simulink model "tank2"  (Simulink 7.3)
settings: Solver=ode45  StartTime=0.0  StopTime=20.0  RelTol=1e-3
undefined symbols (not defined in the file or in its folder): DiscIntNeverNeededParam
libraries: simulink x1
settings Model: Creator=nmd01  LastModifiedBy=nmd01

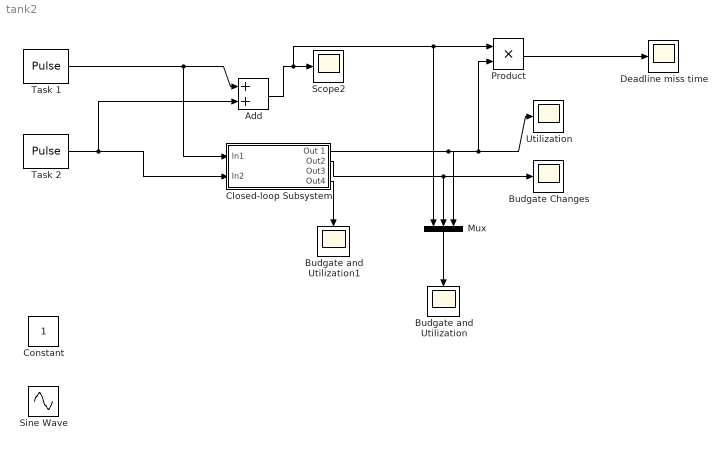
== system tank2 ==
  Add : Sum  OutDataType=fixdt(1, 16)  OutScaling=2^-10
  Budgate Changes : Scope
  Budgate and Utilization : Scope
      settings: TimeRange=200  YMin=0  YMax=30  SaveName=ScopeData3
  Budgate and Utilization1 : Scope
      settings: TimeRange=200  YMin=0  YMax=30
  Closed-loop Subsystem : Subsystem
  Constant : Constant  OutDataType=fixdt(1, 16)  OutScaling=2^0  SampleTime=1
  Deadline miss time : Scope
      settings: SaveName=Sin  DataFormat=Array
  Mux : Mux  Inputs=3
  Product : Product  OutDataType=fixdt(1, 16)  OutScaling=2^0  RndMeth=Zero
  Scope2 : Scope
      settings: SaveName=Sin1  DataFormat=Array
  Sine Wave : Sin  Amplitude=1  Bias=0  Frequency=1  Phase=0  Samples=10  SampleTime=5  Offset=0
  Task 1 : DiscretePulseGenerator  PulseType=Time based  Amplitude=3  Period=5  PulseWidth=1  PhaseDelay=0  SampleTime=1
  Task 2 : DiscretePulseGenerator  PulseType=Time based  Amplitude=2  Period=10  PulseWidth=1  PhaseDelay=0  SampleTime=1
  Utilization : Scope
      settings: SaveName=Utilization  DataFormat=Array
  wires:
  Closed-loop Subsystem/2(Out2) -> Budgate Changes/1, Mux/2
  Mux/1 -> Budgate and Utilization/1
  Task 1/1 -> Closed-loop Subsystem/1(In1), Add/1
  Product/1 -> Deadline miss time/1
  Task 2/1 -> Closed-loop Subsystem/2(In2), Add/2
  Add/1 -> Scope2/1, Product/1, Mux/1
  Closed-loop Subsystem/1(Out 1) -> Utilization/1, Product/2, Mux/3
  Closed-loop Subsystem/4(Out4) -> Budgate and Utilization1/1

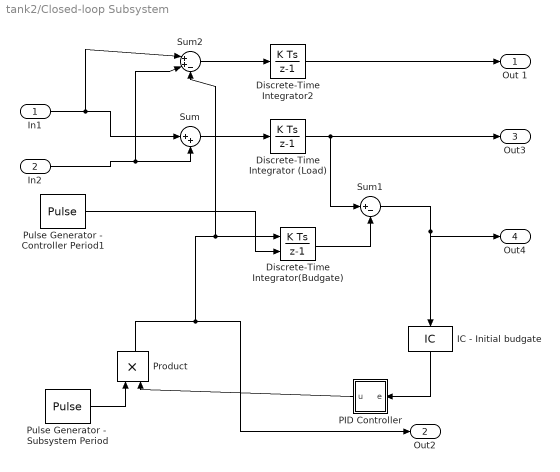
== system tank2/Closed-loop Subsystem ==
  In1 : Inport  OutDataType=fixdt(1, 16)  OutScaling=2^0
  In2 : Inport  Port=2  OutDataType=fixdt(1, 16)  OutScaling=2^0
  Discrete-Time Integrator (Load) : DiscreteIntegrator  OutDataType=fixdt(1, 16)  OutScaling=2^0  LowerSaturationLimit=0  ICPrevOutput=DiscIntNeverNeededParam  ICPrevScaledInput=DiscIntNeverNeededParam
  Discrete-Time Integrator(Budgate) : DiscreteIntegrator  ExternalReset=rising  OutDataType=fixdt(1, 16)  OutScaling=2^0  LowerSaturationLimit=0  ICPrevOutput=DiscIntNeverNeededParam  ICPrevScaledInput=DiscIntNeverNeededParam
  Discrete-Time Integrator2 : DiscreteIntegrator  OutDataType=fixdt(1, 16)  OutScaling=2^0  LimitOutput=on  LowerSaturationLimit=0  ICPrevOutput=DiscIntNeverNeededParam  ICPrevScaledInput=DiscIntNeverNeededParam
  IC - Initial budgate : InitialCondition  Value=2  SampleTime=1
  PID Controller : Subsystem  AncestorBlock=simulink_extras/Additional Linear/PID Controller  mask(PID Controller){P=1, I=.1, D=0}
      mask prompts: P "Proportional:"; I "Integral:"; D "Derivative:"
      mask help:
      | Enter expressions for proportional, integral, and derivative terms.
      | P+I/s+Ds
      mask Help: This block implements a PID controller where parameters are entered for the Proportional, Integral and Derivative terms. Unmask this block to see how it works. The derivative term is implemented using a true derivative block.
      mask Display: disp('PID')
  Product : Product  OutDataType=fixdt(1, 16)  OutScaling=2^0  SampleTime=1  RndMeth=Zero
  Pulse Generator -  Subsystem Period : DiscretePulseGenerator  PulseType=Time based  Amplitude=1  Period=2  PulseWidth=1  PhaseDelay=0  SampleTime=1
  Pulse Generator - Controller Period1 : DiscretePulseGenerator  PulseType=Time based  Amplitude=1  Period=6  PulseWidth=1  PhaseDelay=0  SampleTime=1
  Sum : Sum  Inputs=|++  OutDataType=fixdt(1, 16)  OutScaling=2^0  SampleTime=1
  Sum1 : Sum  Inputs=|+-  OutDataType=fixdt(1, 16)  OutScaling=2^0  SampleTime=6
  Sum2 : Sum  Inputs=|++-  OutDataType=fixdt(1, 16)  OutScaling=2^0  SampleTime=1
  Out 1 : Outport  OutDataType=fixdt(1, 16)  OutScaling=2^0
  Out2 : Outport  Port=2  OutDataType=fixdt(1, 16)  OutScaling=2^0
  Out3 : Outport  Port=3  OutDataType=fixdt(1, 16)  OutScaling=2^0
  Out4 : Outport  Port=4  OutDataType=fixdt(1, 16)  OutScaling=2^0
  wires:
  Discrete-Time Integrator (Load)/1 -> Out3/1, Sum1/1
  In1/1 -> Sum/1, Sum2/1
  Sum/1 -> Discrete-Time Integrator (Load)/1
  PID Controller/1(u) -> Product/2
  Pulse Generator -  Subsystem Period/1 -> Product/1
  Product/1 -> Out2/1, Discrete-Time Integrator(Budgate)/1, Sum2/3
  IC - Initial budgate/1 -> PID Controller/1(e)
  In2/1 -> Sum/2, Sum2/2
  Pulse Generator - Controller Period1/1 -> Discrete-Time Integrator(Budgate)/2
  Discrete-Time Integrator(Budgate)/1 -> Sum1/2
  Sum1/1 -> IC - Initial budgate/1, Out4/1
  Sum2/1 -> Discrete-Time Integrator2/1
  Discrete-Time Integrator2/1 -> Out 1/1

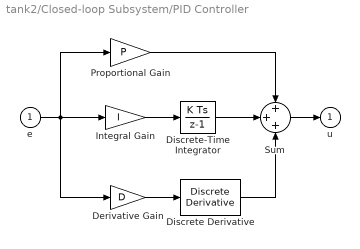
== system tank2/Closed-loop Subsystem/PID Controller ==
  e : Inport  OutDataType=sfix(16)  OutScaling=2^0
  Derivative Gain : Gain  Gain=D  ParameterDataType=sfix(16)  ParameterScaling=2^0  OutDataType=sfix(16)  OutScaling=2^0  SampleTime=6  SaturateOnIntegerOverflow=on  OutDataTypeStr=Inherit: Same as input  ParamDataTypeStr=Inherit: Same as input
  Discrete Derivative : simulink/Discrete/Discrete Derivative  SystemSampleTime=-1  gainval=1.0  ICPrevScaledInput=0.0  OutMin=[]  OutMax=[]  OutDataType=fixdt(1, 16)  OutScaling=2^-10  DoSatur=off
  Discrete-Time Integrator : DiscreteIntegrator  SampleTime=6  OutDataType=fixdt(1, 16)  OutScaling=2^0  ICPrevOutput=DiscIntNeverNeededParam  ICPrevScaledInput=DiscIntNeverNeededParam
  Integral Gain : Gain  Gain=I  ParameterDataType=sfix(16)  ParameterScaling=2^0  OutDataType=sfix(16)  OutScaling=2^0  SampleTime=6  SaturateOnIntegerOverflow=on  OutDataTypeStr=Inherit: Same as input  ParamDataTypeStr=Inherit: Same as input
  Proportional Gain : Gain  Gain=P  ParameterDataType=sfix(16)  ParameterScaling=2^0  OutDataType=sfix(16)  OutScaling=2^0  SampleTime=6  SaturateOnIntegerOverflow=on  OutDataTypeStr=Inherit: Same as input  ParamDataTypeStr=Inherit: Same as input
  Sum : Sum  Inputs=+++  OutDataType=sfix(16)  OutScaling=2^0  SaturateOnIntegerOverflow=on  InputSameDT=on  OutDataTypeStr=Inherit: Same as first input
  u : Outport  OutDataType=sfix(16)  OutScaling=2^0  InitialOutput=0
  wires:
  Integral Gain/1 -> Discrete-Time Integrator/1
  Proportional Gain/1 -> Sum/1
  Discrete-Time Integrator/1 -> Sum/2
  Discrete Derivative/1 -> Sum/3
  e/1 -> Derivative Gain/1, Proportional Gain/1, Integral Gain/1
  Sum/1 -> u/1
  Derivative Gain/1 -> Discrete Derivative/1
